simulink model "OFDMTxRx2211221"  (R2017b)
settings: Solver=VariableStepAuto  StartTime=0.0  StopTime=10  RelTol=1e-3
InitFcn:
  | Ts = 1e-6;
  | simParams.Ts = Ts;
  | simParams.TsTx = Ts;
  | simParams.TsRx = Ts;
  | simParams.nFFT = 1024;
  | simParams.lengthCP = 128;
  | nFFT = simParams.nFFT;
  | simParams.NSubcarriers = 398;
  | simParams.windowing = 16;
undefined symbols (not defined in the file): fft_size, i
libraries: hdlsllib x35, simulink x28, simulink_need_slupdate x17, dspmathops x5, dspxfrm3 x3, dspsigops x2, commdigbbndam3 x1, commrflib2 x1, commseqgen3 x1
(part 3 of 3)

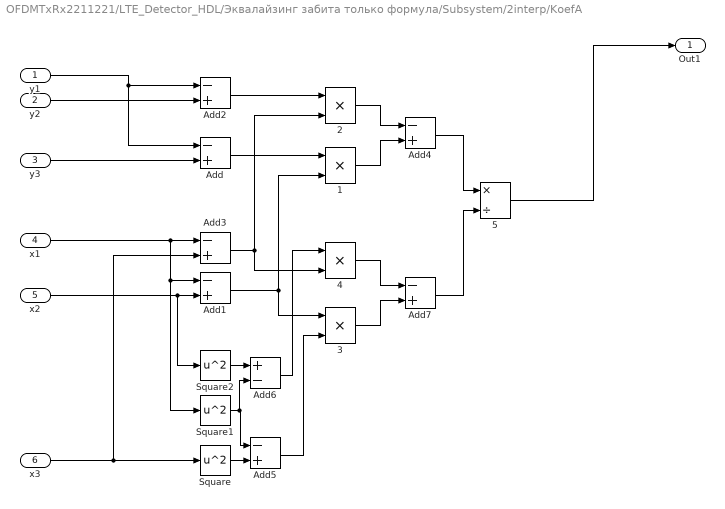
== system OFDMTxRx2211221/LTE_Detector_HDL/Эквалайзинг забита только формула/Subsystem/2interp/KoefA  ==
  y1 : Inport
  y2 : Inport  Port=2
  y3 : Inport  Port=3
  x1 : Inport  Port=4
  x2 : Inport  Port=5
  x3 : Inport  Port=6
  {1..4} (4 alike) : Product  Inputs=**  SaturateOnIntegerOverflow=on  RndMeth=Zero
  5 : Product  Inputs=*/  SaturateOnIntegerOverflow=on  RndMeth=Zero
  Add{,1..5,7} (7 alike) : Sum  Inputs=-+
  Add6 : Sum  Inputs=+-
  Square : Math  Operator=square  RndMeth=Zero  SaturateOnIntegerOverflow=on
  Square1 : Math  Operator=square  RndMeth=Zero  SaturateOnIntegerOverflow=on
  Square2 : Math  Operator=square  RndMeth=Zero  SaturateOnIntegerOverflow=on
  Out1 : Outport
  wires:
  Add/1 -> 1/1
  5/1 -> Out1/1
  Add5/1 -> 3/2
  x1/1 -> Square1/1, Add1/1, Add3/1
  3/1 -> Add7/2
  Add4/1 -> 5/1
  x3/1 -> Add3/2, Square/1
  Add7/1 -> 5/2
  Add2/1 -> 2/1
  4/1 -> Add7/1
  y2/1 -> Add2/2
  Square1/1 -> Add6/2, Add5/1
  Square2/1 -> Add6/1
  2/1 -> Add4/1
  Add1/1 -> 3/1, 1/2
  1/1 -> Add4/2
  Add3/1 -> 4/2, 2/2
  y3/1 -> Add/2
  y1/1 -> Add2/1, Add/1
  Add6/1 -> 4/1
  x2/1 -> Square2/1, Add1/2
  Square/1 -> Add5/2

== system OFDMTxRx2211221/LTE_Detector_HDL/Эквалайзинг забита только формула/Subsystem/2interp/Subsystem ==
  y1 : Inport
  "y2 " : Inport  Port=2
  a : Inport  Port=3
  x1 : Inport  Port=4
  "x2 " : Inport  Port=5
  1 : Product  Inputs=**  SaturateOnIntegerOverflow=on  RndMeth=Zero
  2 : Product  Inputs=/*  SaturateOnIntegerOverflow=on  RndMeth=Zero
  Add1 : Sum  Inputs=+-
  Add2 : Sum  Inputs=+--
  Add3 : Sum  Inputs=+-
  Square : Math  Operator=square  RndMeth=Zero  SaturateOnIntegerOverflow=on
  Square1 : Math  Operator=square  RndMeth=Zero  SaturateOnIntegerOverflow=on
  b : Outport
  wires:
  1/1 -> Add2/3
  Square1/1 -> Add1/1
  Add2/1 -> 2/2
  "x2 "/1 -> Add3/1, Square1/1
  y1/1 -> Add2/2
  "y2 "/1 -> Add2/1
  a/1 -> 1/1
  2/1 -> b/1
  x1/1 -> Add3/2, Square/1
  Add1/1 -> 1/2
  Square/1 -> Add1/2
  Add3/1 -> 2/1

== system OFDMTxRx2211221/LTE_Detector_HDL/Эквалайзинг забита только формула/Subsystem/2interp/Subsystem1 ==
  y1 : Inport
  a : Inport  Port=2
  b : Inport  Port=3
  x1 : Inport  Port=4
  1 : Product  Inputs=**  SaturateOnIntegerOverflow=on  RndMeth=Zero
  2 : Product  Inputs=**  SaturateOnIntegerOverflow=on  RndMeth=Zero
  Add1 : Sum  Inputs=+--
  Square1 : Math  Operator=square  RndMeth=Zero  SaturateOnIntegerOverflow=on
  c : Outport
  wires:
  Square1/1 -> 1/2
  1/1 -> Add1/3
  Add1/1 -> c/1
  a/1 -> 1/1
  x1/1 -> Square1/1, 2/2
  b/1 -> 2/1
  y1/1 -> Add1/1
  2/1 -> Add1/2
